simulink model "EV"  (R2021b)
settings: Solver=ode1  StartTime=0.0  StopTime=1180*18  FixedStep=0.1  RelTol=1e-3
values from neighbouring files (symbols this model uses):
  A = 1.97    [vehicle_init.m]
  Cd = 0.29    [vehicle_init.m]
  g = 9.8    [vehicle_init.m]
  i = 6.058    [vehicle_init.m]
  n = 0.95    [vehicle_init.m]
  r = 0.334    [vehicle_init.m]
  Vehicle_Mass = 1700    [vehicle_init.m]
undefined symbols (not defined in the file or in its folder): Mot_drive_n, Mot_drive_ttq, Mot_eff
libraries: autolibshared x1
settings Model: Creator=atong  LastModifiedBy=atong

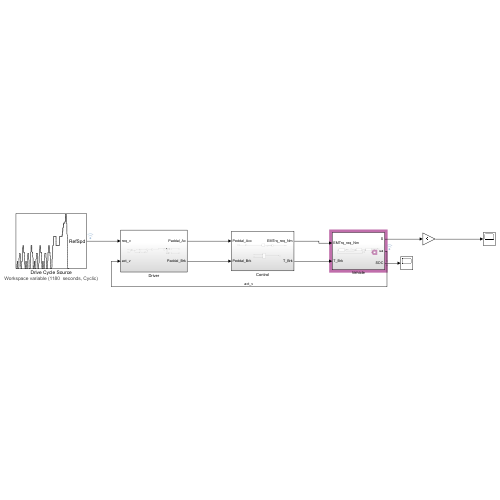
[thumbnail: Simulink's stored preview of the top-level diagram]
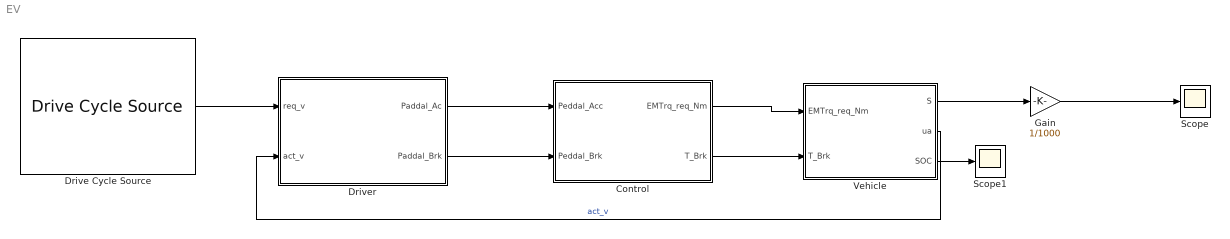
== system EV ==
  Control : Subsystem
  Drive Cycle Source : autolibshared/Drive Cycle Source  cycleVar=Workspace variable  wsVar=sch_cycle  fileVar=cycleFTP75.mat  tfinal="1180  seconds, Cyclic"  cycleRepeat=on  outAccPort=off  outGearPort=off  gearList=No gear data  t_wot1=5  xdot_woto=0  xdot_wot1=30  t_wot2=20  xdot_wot2=0  t_wotend=30  srcUnit=m/s  outUnit=m/s  srcAccUnit=m/s/s  outAccUnit=m/s^2  dt=0  aMode=1  faultOption=off  velBnd=2  velBndUnit=mph  inUnit=m/s  timeBnd=1  failOption=off  stopSim=off  maxFaultCnt=10  maxFaultTime=2  maxTotFaultTime=15  traceOption=off  dtTrace=1  traceWindow=10  lastDCname=Custom Data Set  lastOutUnit=mph  lastDT=0  lastTB=1  lastSB=2  forceCalcBound=off
      settings: SourceProductBaseCode=PW,DR,MT,UV,VE
  Driver : Subsystem
  Gain : Gain  Gain=1/1000
  Scope : Scope
  Scope1 : Scope
  Vehicle : Subsystem
  wires:
  Control/1(EMTrq_req_Nm) -> Vehicle/1(EMTrq_req_Nm)
  Driver/1(Paddal_Ac) -> Control/1(Peddal_Acc)
  Driver/2(Paddal_Brk) -> Control/2(Peddal_Brk)
  Control/2(T_Brk) -> Vehicle/2(T_Brk)
  Vehicle/2(ua) -> Driver/2(act_v)  "act_v"
  Vehicle/1(S) -> Gain/1
  Vehicle/3(SOC) -> Scope1/1
  Drive Cycle Source/1 -> Driver/1(req_v)
  Gain/1 -> Scope/1

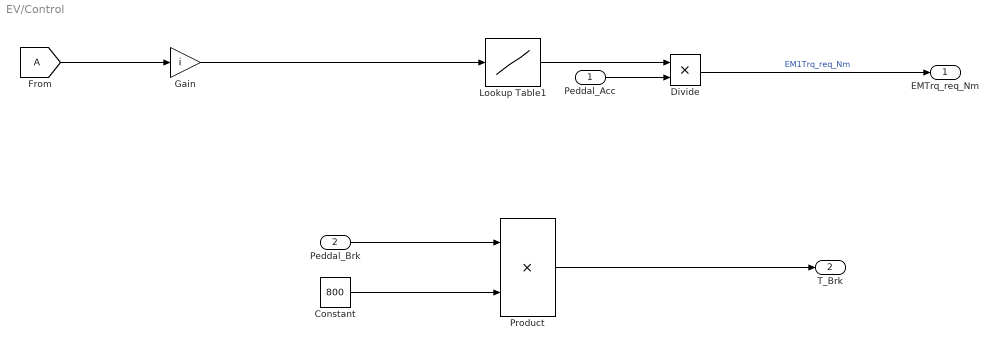
== system EV/Control ==
  Peddal_Acc : Inport
  Peddal_Brk : Inport  Port=2
  Constant : Constant  Value=800
  Divide : Product  Inputs=**
  Gain : Gain  Gain=i
  Lookup Table1 : Lookup  InputValues=Mot_drive_n  Table=Mot_drive_ttq
  Product : Product
  EMTrq_req_Nm : Outport
  T_Brk : Outport  Port=2
  wires:
  Gain/1 -> Lookup Table1/1
  Divide/1 -> EMTrq_req_Nm/1  "EM1Trq_req_Nm"
  Lookup Table1/1 -> Divide/1
  Peddal_Acc/1 -> Divide/2
  [A] -> Gain/1
  Peddal_Brk/1 -> Product/1
  Constant/1 -> Product/2
  Product/1 -> T_Brk/1

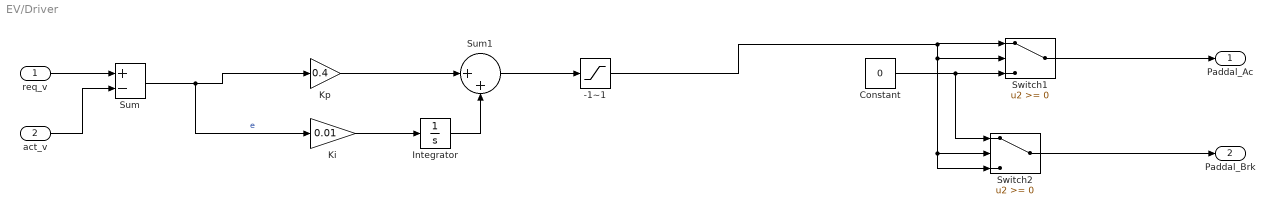
== system EV/Driver ==
  req_v : Inport
  act_v : Inport  Port=2
  -1~1 : Saturate  UpperLimit=1  LowerLimit=-1
  Constant : Constant  Value=0
  Integrator : Integrator
  Ki : Gain  Gain=0.01
  Kp : Gain  Gain=0.4
  Sum : Sum  Inputs=+-
  Sum1 : Sum  Inputs=|++
  Switch1 : Switch
  Switch2 : Switch
  Paddal_Ac : Outport
  Paddal_Brk : Outport  Port=2
  wires:
  Constant/1 -> Switch2/1, Switch1/3
  Switch2/1 -> Paddal_Brk/1
  Switch1/1 -> Paddal_Ac/1
  -1~1/1 -> Switch2/3, Switch2/2, Switch1/2, Switch1/1
  Integrator/1 -> Sum1/2
  Ki/1 -> Integrator/1
  Sum1/1 -> -1~1/1
  Kp/1 -> Sum1/1
  req_v/1 -> Sum/1
  act_v/1 -> Sum/2
  Sum/1 -> Ki/1, Kp/1  "e"

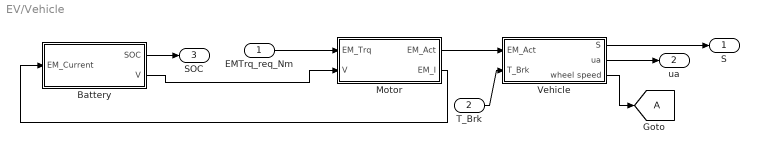
== system EV/Vehicle ==
  EMTrq_req_Nm : Inport
  T_Brk : Inport  Port=2
  Battery : Subsystem
  Motor : Subsystem
  Vehicle : Subsystem
  S : Outport
  ua : Outport  Port=2
  SOC : Outport  Port=3
  tag scope: A=global
  wires:
  Battery/2(V) -> Motor/2(V)
  Motor/2(EM_I) -> Battery/1(EM_Current)
  EMTrq_req_Nm/1 -> Motor/1(EM_Trq)
  Motor/1(EM_Act) -> Vehicle/1(EM_Act)
  T_Brk/1 -> Vehicle/2(T_Brk)
  Vehicle/1(S) -> S/1
  Vehicle/2(ua) -> ua/1
  Battery/1(SOC) -> SOC/1
  Vehicle/3(wheel speed) -> [A]

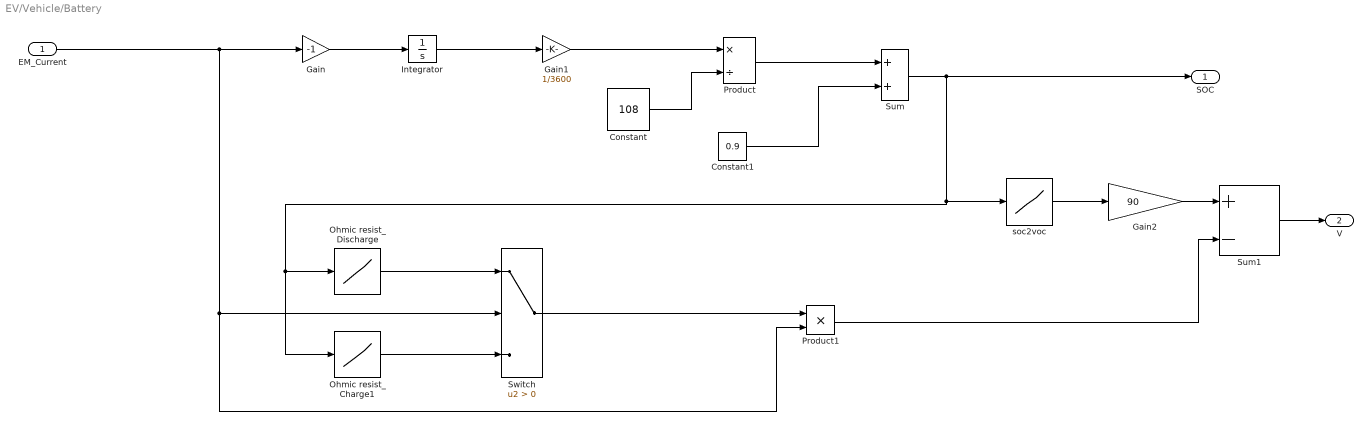
== system EV/Vehicle/Battery ==
  EM_Current : Inport
  Constant : Constant  Value=108
  Constant1 : Constant  Value=0.9
  Gain : Gain  Gain=-1
  Gain1 : Gain  Gain=1/3600
  Gain2 : Gain  Gain=90
  Integrator : Integrator
  Ohmic resist_Charge1 : Lookup  InputValues=[0,0.1,0.2,0.4,0.6,0.8,1]  Table=[0.02536,0.012695,0.0080907,0.006409000000000001,0.006565,0.0071812,0.0074386]
  Ohmic resist_Discharge : Lookup  InputValues=[0,0.1,0.2,0.4,0.6,0.8,1]  Table=[0.02536,0.012695,0.0080907,0.006409000000000001,0.006565,0.0071812,0.0074386]
  Product : Product  Inputs=*/
  Product1 : Product
  Sum : Sum
  Sum1 : Sum  Inputs=+-
  Switch : Switch  Criteria=u2 > Threshold
  soc2voc : Lookup  InputValues=[0,0.1,0.2,0.4,0.6,0.8,1]  Table=[3.31144,3.54994000000000013,3.63898,3.72908,3.8329600000000004,3.9771199999999998,4.131880000000001]
  SOC : Outport
  V : Outport  Port=2
  wires:
  EM_Current/1 -> Switch/2, Product1/2, Gain/1
  Gain/1 -> Integrator/1
  Integrator/1 -> Gain1/1
  Gain1/1 -> Product/1
  Constant/1 -> Product/2
  Product/1 -> Sum/1
  Constant1/1 -> Sum/2
  Sum/1 -> SOC/1, Ohmic resist_Charge1/1, Ohmic resist_Discharge/1, soc2voc/1
  Ohmic resist_Charge1/1 -> Switch/3
  Ohmic resist_Discharge/1 -> Switch/1
  Switch/1 -> Product1/1
  soc2voc/1 -> Gain2/1
  Gain2/1 -> Sum1/1
  Product1/1 -> Sum1/2
  Sum1/1 -> V/1

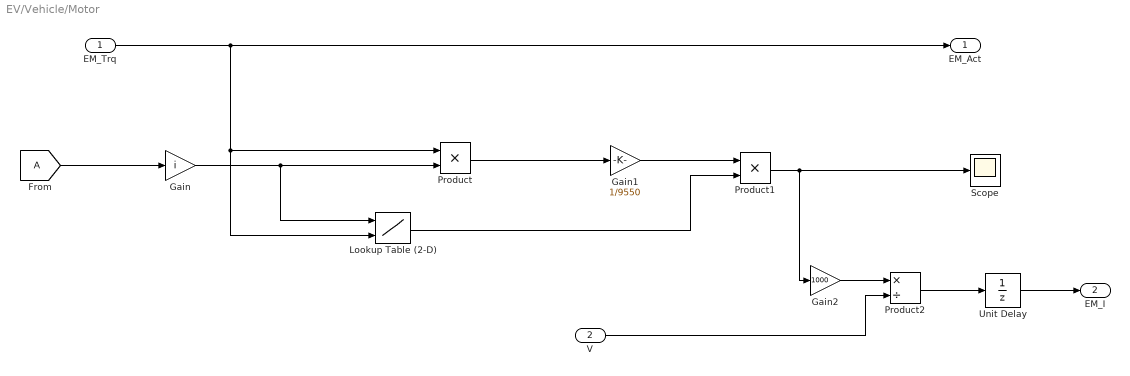
== system EV/Vehicle/Motor ==
  EM_Trq : Inport
  V : Inport  Port=2
  Gain : Gain  Gain=i
  Gain1 : Gain  Gain=1/9550
  Gain2 : Gain  Gain=1000
  Lookup Table (2-D) : Lookup2D  RowIndex="[500,1000\t,2000,3200,4000,5000,6000,7000,8000,9000,10000]"  ColumnIndex=[30,60,92,120,150,180]  Table=Mot_eff  LookUpMeth=Interpolation-Use End Values
  Product : Product
  Product1 : Product
  Product2 : Product  Inputs=*/
  Scope : Scope
  Unit Delay : UnitDelay  SampleTime=-1  HasFrameUpgradeWarning=on
  EM_Act : Outport
  EM_I : Outport  Port=2
  wires:
  EM_Trq/1 -> Lookup Table (2-D)/2, Product/1, EM_Act/1
  [A] -> Gain/1
  Gain/1 -> Lookup Table (2-D)/1, Product/2
  Product/1 -> Gain1/1
  Gain1/1 -> Product1/1
  Lookup Table (2-D)/1 -> Product1/2
  Product1/1 -> Gain2/1, Scope/1
  Gain2/1 -> Product2/1
  V/1 -> Product2/2
  Product2/1 -> Unit Delay/1
  Unit Delay/1 -> EM_I/1

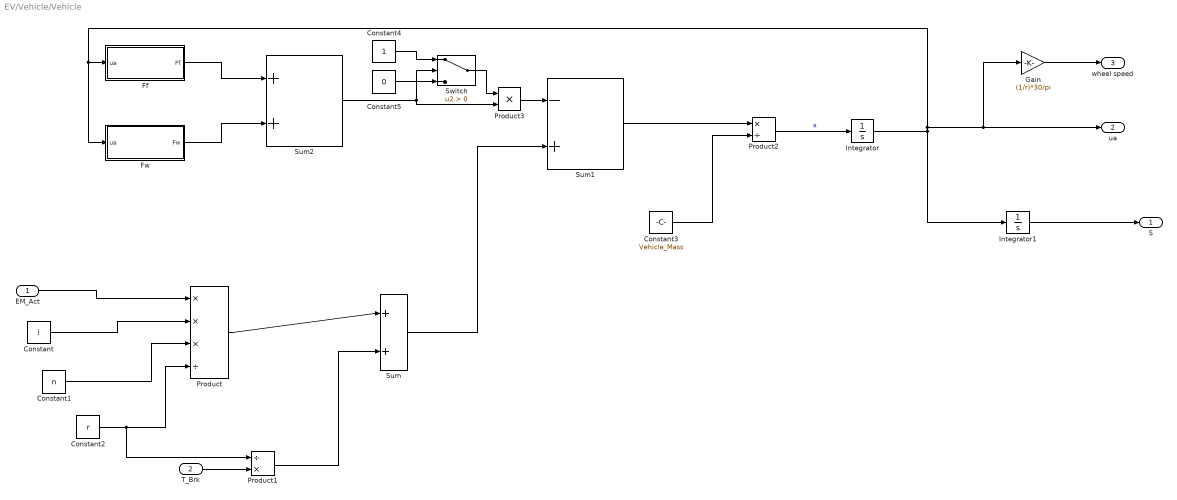
== system EV/Vehicle/Vehicle ==
  EM_Act : Inport
  T_Brk : Inport  Port=2
  Constant : Constant  Value=i
  Constant1 : Constant  Value=n
  Constant2 : Constant  Value=r
  Constant3 : Constant  Value=Vehicle_Mass
  Constant4 : Constant
  Constant5 : Constant  Value=0
  Ff : Subsystem
  Fw : Subsystem
  Gain : Gain  Gain=(1/r)*30/pi
  Integrator : Integrator
  Integrator1 : Integrator
  Product : Product  Inputs=***/
  Product1 : Product  Inputs=/*
  Product2 : Product  Inputs=*/
  Product3 : Product
  Sum : Sum  Inputs=|++
  Sum1 : Sum  Inputs=-+
  Sum2 : Sum
  Switch : Switch  Criteria=u2 > Threshold
  S : Outport
  ua : Outport  Port=2
  wheel speed : Outport  Port=3
  wires:
  EM_Act/1 -> Product/1
  Constant/1 -> Product/2
  Constant1/1 -> Product/3
  Constant2/1 -> Product/4, Product1/1
  T_Brk/1 -> Product1/2
  Product/1 -> Sum/1
  Product1/1 -> Sum/2
  Ff/1(Ff) -> Sum2/1
  Fw/1(Fw) -> Sum2/2
  Sum/1 -> Sum1/2
  Sum1/1 -> Product2/1
  Constant3/1 -> Product2/2
  Product2/1 -> Integrator/1  "a"
  Integrator1/1 -> S/1
  Gain/1 -> wheel speed/1
  Integrator/1 -> Gain/1, ua/1, Fw/1(ua), Ff/1(ua), Integrator1/1
  Sum2/1 -> Switch/2, Product3/2
  Constant5/1 -> Switch/3
  Constant4/1 -> Switch/1
  Product3/1 -> Sum1/1
  Switch/1 -> Product3/1

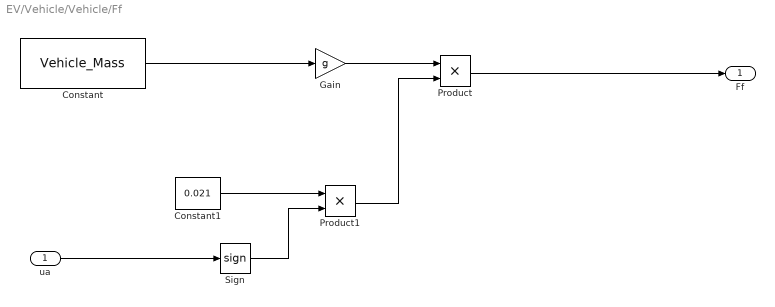
== system EV/Vehicle/Vehicle/Ff ==
  ua : Inport
  Constant : Constant  Value=Vehicle_Mass
  Constant1 : Constant  Value=0.021
  Gain : Gain  Gain=g
  Product : Product
  Product1 : Product
  Sign : Signum
  Ff : Outport
  wires:
  Constant/1 -> Gain/1
  Gain/1 -> Product/1
  Product/1 -> Ff/1
  ua/1 -> Sign/1
  Constant1/1 -> Product1/1
  Sign/1 -> Product1/2
  Product1/1 -> Product/2

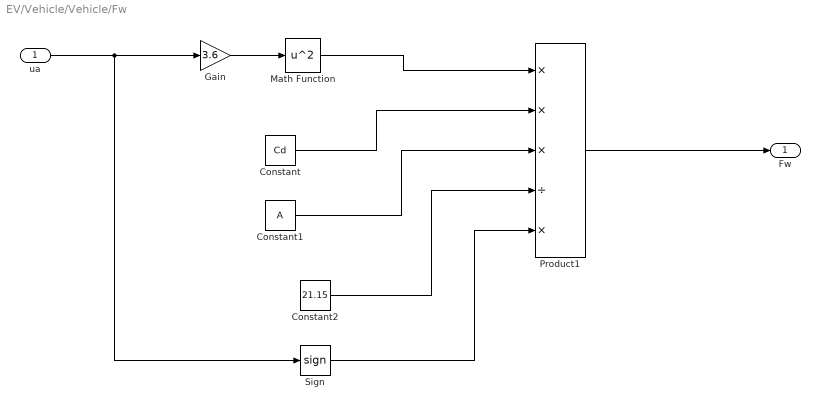
== system EV/Vehicle/Vehicle/Fw ==
  ua : Inport
  Constant : Constant  Value=Cd
  Constant1 : Constant  Value=A
  Constant2 : Constant  Value=21.15
  Gain : Gain  Gain=3.6
  Math Function : Math  Operator=square  SaturateOnIntegerOverflow=on
  Product1 : Product  Inputs=***/*
  Sign : Signum
  Fw : Outport
  wires:
  ua/1 -> Sign/1, Gain/1
  Math Function/1 -> Product1/1
  Constant/1 -> Product1/2
  Constant1/1 -> Product1/3
  Constant2/1 -> Product1/4
  Product1/1 -> Fw/1
  Gain/1 -> Math Function/1
  Sign/1 -> Product1/5
